simulink model "PAM_SIM"  (R2024a)
settings: Solver=VariableStepAuto  StartTime=0.0  StopTime=10.0  RelTol=1e-3
libraries: dspfdesign x1, simulink x1, spsMonostableLib x1
settings Model: Creator=adity  LastModifiedBy=adity

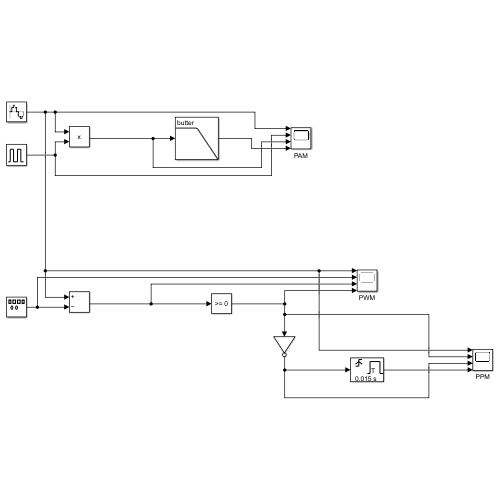
[thumbnail: Simulink's stored preview of the top-level diagram]
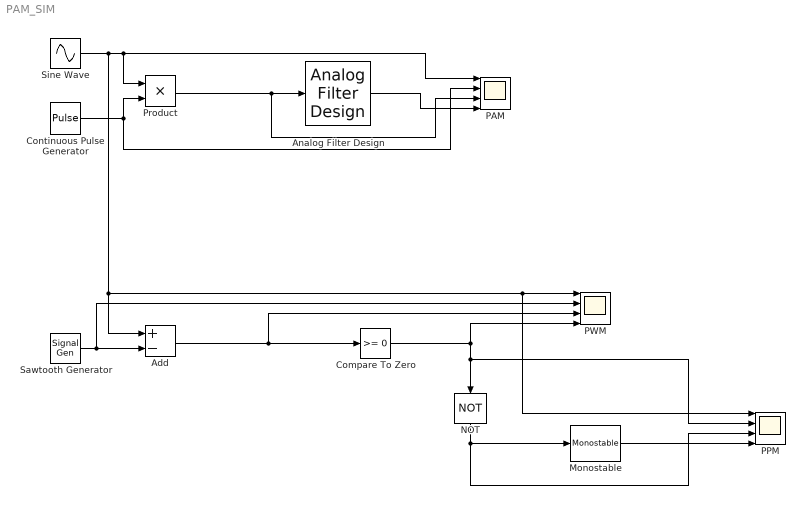
== system PAM_SIM ==
  Add : Sum  Inputs=+-
  Analog Filter Design : dspfdesign/Analog Filter Design  method=Butterworth  filttype=Lowpass  N=8  Wlo=30  Whi=80  Rp=2  Rs=40
  Compare To Zero : simulink/Logic and Bit Operations/Compare To Zero  relop=>=  OutDataTypeStr=boolean
  Continuous Pulse Generator : DiscretePulseGenerator  PulseType=Time based  Period=0.02  PulseWidth=50
  Monostable : spsMonostableLib/Monostable  EdgeDetect=Rising  PulseDuration=0.015  ic=0  Ts=0
      settings: LibrarySourceBlock=sps_lib/Control/Monostable
  NOT : Logic  Operator=NOT  IconShape=distinctive  AllPortsSameDT=off  OutDataTypeStr=boolean
  PAM : Scope  NumInputPorts=4
  PPM : Scope  NumInputPorts=4
  PWM : Scope  NumInputPorts=4
  Product : Product
  Sawtooth Generator : SignalGenerator  WaveForm=sawtooth  Frequency=10
  Sine Wave : Sin  Frequency=2*pi*1  SampleTime=1/1000
  wires:
  Sine Wave/1 -> Add/1, PPM/1, PWM/1, PAM/1, Product/1
  Continuous Pulse Generator/1 -> PAM/2, Product/2
  Product/1 -> PAM/3, Analog Filter Design/1
  Analog Filter Design/1 -> PAM/4
  Sawtooth Generator/1 -> PWM/2, Add/2
  Add/1 -> PWM/3, Compare To Zero/1
  Compare To Zero/1 -> PWM/4, PPM/2, NOT/1
  NOT/1 -> Monostable/1, PPM/3
  Monostable/1 -> PPM/4
